simulink model "dualSpinCSSimulink"  (R2022a)
settings: Solver=VariableStepAuto  StartTime=0.0  StopTime=200  RelTol=1e-3
values from neighbouring files (symbols this model uses):
  alpha = 0.9    [dualSpinControlSystem.m]
  h_dot = 0    [dualSpinControlSystem.m]
  h_s = I_B * w_B    [dualSpinControlSystem.m]
  Ixx = 44451.50    (= 44451.5)    [dualSpinControlSystem.m]    (also in nonlinear_linear.m = interiaVector(1); singleSpinSystem.m)
  Iyy = 45161.45    [dualSpinControlSystem.m]    (also in nonlinear_linear.m = interiaVector(2); singleSpinSystem.m)
  Izz = 44017.00    (= 44017)    [dualSpinControlSystem.m]    (also in nonlinear_linear.m = interiaVector(3); singleSpinSystem.m)
  kd = 1.2    [dualSpinControlSystem.m]
  kd_p = 2 * Iyy * zeta_pitch * wN_pitch    [dualSpinControlSystem.m]
  kg = 3 * w_0_b2^2 * (Ixx-Izz)    [dualSpinControlSystem.m]
  kp = 3    [dualSpinControlSystem.m]
  kp_p = wN_pitch^2*Iyy - 3*w_0_b2^2 * (Ixx - Izz)    [dualSpinControlSystem.m]
  T = 5    [dualSpinControlSystem.m]
  tC_x = 0    [dualSpinControlSystem.m]
  tC_y = 0    [dualSpinControlSystem.m]
  tC_z = 0    [dualSpinControlSystem.m]
  tD_x = 1E-5    (= 1e-05)    [dualSpinControlSystem.m]
  tD_y = 1E-5    (= 1e-05)    [dualSpinControlSystem.m]
  tD_z = 1E-5    (= 1e-05)    [dualSpinControlSystem.m]
  w_0_b2 = sqrt(mu/R_c^3)    [dualSpinControlSystem.m]
undefined symbols (not defined in the file or in its folder): ki
settings Model: Creator=micha  LastModifiedBy=micha

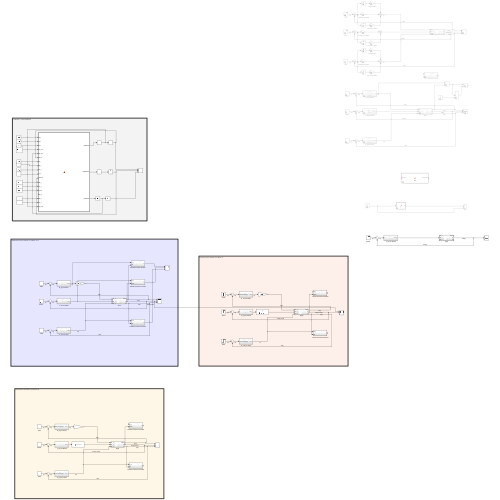
[thumbnail: Simulink's stored preview of the top-level diagram]
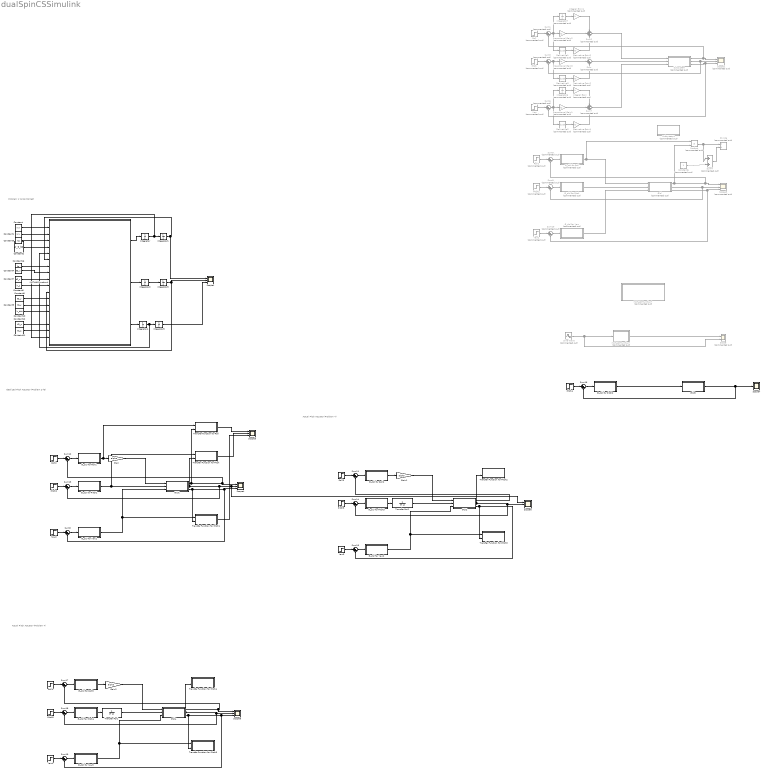
== system dualSpinCSSimulink ==
  note: Problem 1 (Uncontrolled)
  note: Actual Pitch Actuator (Problem 4)
  note: Idealized Pitch Actuator (Problem 2+3)
  note: Actual Pitch Actuator (Problem 4)
  Constant : Constant  Value=Ixx
  Constant1 : Constant  Value=Iyy
  Constant10 : Constant  Value=h_dot
  Constant11 : Constant  Value=tC_z
  Constant12 : Constant  Value=tD_z
  Constant16 : Constant  Value=kg
  Constant2 : Constant  Value=w_0_b2
  Constant3 : Constant  Value=Izz
  Constant4 : Constant  Value=tD_x
  Constant5 : Constant  Value=h_s
  Constant6 : Constant  Commented=on
  Constant7 : Constant  Value=tC_x
  Constant8 : Constant  Value=tD_y
  Constant9 : Constant  Value=tC_y
  Derivative Gain1 : Gain  Commented=on  Gain=kd
  Derivative Gain2 : Gain  Commented=on  Gain=kd
  Derivative Gain3 : Gain  Commented=on  Gain=kd
  Derivative1 : Derivative  Commented=on
  Derivative2 : Derivative  Commented=on
  Derivative3 : Derivative  Commented=on
  Divide : Product  Commented=on  Inputs=*/
  G(s) : Subsystem  Commented=on
  G(s)1 : Subsystem
  G(s)2 : Subsystem
  G(s)3 : Subsystem
  G(s)4 : Subsystem
  G_c(s) for Pitch : Subsystem  Commented=on
  G_c(s) for Pitch1 : Subsystem
  G_c(s) for Pitch2 : Subsystem
  G_c(s) for Pitch3 : Subsystem
  G_c(s) for Pitch4 : Subsystem
  G_c(s) for Roll : Subsystem  Commented=on
  G_c(s) for Roll1 : Subsystem
  G_c(s) for Roll2 : Subsystem
  G_c(s) for Roll3 : Subsystem
  G_c(s) for Yaw : Subsystem  Commented=on
  G_c(s) for Yaw1 : Subsystem
  G_c(s) for Yaw2 : Subsystem
  G_c(s) for Yaw3 : Subsystem
  Gain : Gain  Gain=alpha
  Gain1 : Gain  Gain=alpha
  Gain2 : Gain  Gain=alpha
  Integral Gain : Gain  Commented=on  Gain=ki
  Integral Gain1 : Gain  Commented=on  Gain=ki
  Integrator{,1..5} (6 alike) : Integrator
  Integrator6 : Integrator  Commented=on
  Integrator7 : Integrator  Commented=on
  MATLAB Function1 : MATLAB Function  Commented=on  TreatAsAtomicUnit=on
  MATLAB Function2 : MATLAB Function  Commented=on  TreatAsAtomicUnit=on
  MATLAB Function4 : MATLAB Function  TreatAsAtomicUnit=on
  Pitch : Step  Commented=on  SampleTime=0
  Pitch1 : Step  Commented=on  SampleTime=0
  Pitch{2..5} (4 alike) : Step  SampleTime=0
  Product : Product  Commented=on
  Proportional Gain1 : Gain  Commented=on  Gain=kp
  Proportional Gain2 : Gain  Commented=on  Gain=kp
  Proportional Gain3 : Gain  Commented=on  Gain=kp
  Roll : Step  Commented=on  SampleTime=0
  Roll1 : Step  Commented=on  SampleTime=0
  Roll2 : Step  SampleTime=0
  Roll3 : Step  SampleTime=0
  Roll4 : Step  SampleTime=0
  Scope : Scope  Commented=on  NumInputPorts=2
  Scope{1,4..8} (6 alike) : Scope  NumInputPorts=3
  Scope2 : Scope  Commented=on  NumInputPorts=3
  Scope3 : Scope  Commented=on  NumInputPorts=3
  Sine Wave : Sin  Commented=on  SampleTime=0
  Subsystem : Subsystem  Commented=on
  Subsystem1 : Subsystem  Commented=on
  Sum : Sum  Commented=on  Inputs=|++
  Sum{1,3,5..6,9..10} (6 alike) : Sum  Commented=on  Inputs=|+-
  Sum{8,11..19} (10 alike) : Sum  Inputs=|+-
  Sum2 : Sum  Commented=on  Inputs=+++
  Sum4 : Sum  Commented=on  Inputs=|++
  Sum7 : Sum  Commented=on  Inputs=+++
  Transfer Fcn1 : TransferFcn  Denominator=[T 1]
  Transfer Fcn2 : TransferFcn  Denominator=[T 1]
  Transfer Function for Pitch : Subsystem
  Transfer Function for Pitch1 : Subsystem
  Transfer Function for Pitch2 : Subsystem
  Transfer Function for Pitch3 : Subsystem
  Transfer Function for Pitch4 : Subsystem
  Transfer Function for Pitch5 : Subsystem
  "Transfer Function for Roll " : Subsystem
  Yaw : Step  Commented=on  SampleTime=0
  Yaw1 : Step  Commented=on  SampleTime=0
  Yaw2 : Step  SampleTime=0
  Yaw3 : Step  SampleTime=0
  Yaw4 : Step  SampleTime=0
  wires:
  MATLAB Function1/1(y) -> Scope/1
  Sine Wave/1 -> Scope/2, MATLAB Function1/1(u)
  MATLAB Function4/1(phiDotDot) -> Integrator/1
  Integrator/1 -> MATLAB Function4/18(phi_dot), Integrator1/1
  Constant/1 -> MATLAB Function4/1(Ixx)
  Constant1/1 -> MATLAB Function4/2(Iyy)
  Constant3/1 -> MATLAB Function4/3(Izz)
  Constant16/1 -> MATLAB Function4/7(kg)
  Constant4/1 -> MATLAB Function4/8(tD_x)
  Constant7/1 -> MATLAB Function4/9(tC_x)
  Constant2/1 -> MATLAB Function4/4(w_0_b2)
  Constant5/1 -> MATLAB Function4/10(h_s)
  Constant8/1 -> MATLAB Function4/12(tD_y)
  Constant9/1 -> MATLAB Function4/13(tC_y)
  Constant10/1 -> MATLAB Function4/14(h_dot)
  Constant12/1 -> MATLAB Function4/16(tD_z)
  Constant11/1 -> MATLAB Function4/17(tC_z)
  Integrator1/1 -> Scope1/1, MATLAB Function4/6(phi_0)
  MATLAB Function4/2(thetaDotDot) -> Integrator2/1
  Integrator2/1 -> Integrator3/1
  Integrator3/1 -> Scope1/2, MATLAB Function4/11(theta_0)
  Integrator4/1 -> MATLAB Function4/5(psi_dot), Integrator5/1
  MATLAB Function4/3(psiDotDot) -> Integrator4/1
  Integrator5/1 -> Scope1/3
  Proportional Gain1/1 -> Sum7/2
  Integrator6/1 -> Integral Gain/1
  Derivative2/1 -> Derivative Gain1/1
  Subsystem/3(Out3) -> Scope2/3, Sum6/2  "psi(t)"
  Yaw/1 -> Sum6/1  "u(t)"
  Sum6/1 -> Derivative2/1, Integrator6/1, Proportional Gain1/1  "e(t)"
  Integral Gain/1 -> Sum7/1
  Derivative Gain1/1 -> Sum7/3
  Sum1/1 -> Derivative1/1, Integrator7/1, Proportional Gain2/1  "e(t)"
  Integral Gain1/1 -> Sum2/1
  Derivative Gain2/1 -> Sum2/3
  Proportional Gain2/1 -> Sum2/2
  Integrator7/1 -> Integral Gain1/1
  Subsystem/1(Out1) -> Sum1/2, Scope2/1  "phi(t)"
  Derivative1/1 -> Derivative Gain2/1
  Roll/1 -> Sum1/1  "u(t)"
  Sum3/1 -> Derivative3/1, Proportional Gain3/1  "e(t)"
  Derivative Gain3/1 -> Sum/2
  Subsystem/2(Out2) -> Sum3/2, Scope2/2  "theta(t)"
  Derivative3/1 -> Derivative Gain3/1
  Pitch/1 -> Sum3/1  "u(t)"
  Proportional Gain3/1 -> Sum/1
  Sum7/1 -> Subsystem/3(tC_z)  "v(t)"
  Sum2/1 -> Subsystem/1(tC_x)  "v(t)"
  Sum/1 -> Subsystem/2(tC_y)
  G_c(s) for Roll/1(Out1) -> Product/1, G(s)/1(tC_x)  "v(t)"
  Sum9/1 -> G_c(s) for Pitch/1(In1)  "e(t)"
  G_c(s) for Yaw/1(tC_z) -> G(s)/3(tC_z)  "v(t)"
  G(s)/2(Out2) -> Sum9/2, Scope3/2  "theta(t)"
  Sum10/1 -> G_c(s) for Yaw/1(In1)  "e(t)"
  Roll1/1 -> Sum5/1  "u(t)"
  G(s)/3(Out3) -> Scope3/3, Sum10/2  "psi(t)"
  Pitch1/1 -> Sum9/1  "u(t)"
  G(s)/1(Out1) -> Product/2, Sum5/2, Scope3/1  "phi(t)"
  Yaw1/1 -> Sum10/1  "u(t)"
  G_c(s) for Pitch/1(tC_y) -> G(s)/2(tC_y)
  Sum5/1 -> G_c(s) for Roll/1(In1)  "e(t)"
  Product/1 -> Sum4/1, Divide/1
  Constant6/1 -> Sum4/2
  Sum4/1 -> Divide/2
  Sum8/1 -> G_c(s) for Yaw1/1(In1)  "e(t)"
  G_c(s) for Yaw1/1(tC_z) -> G(s)1/3(tC_z), Transfer Function for Pitch1/1(tC_z)  "v(t)"
  Yaw2/1 -> Sum8/1  "u(t)"
  G(s)1/1(Input) -> "Transfer Function for Roll "/2(phi), Scope4/1, Sum12/2  "phi(t)"
  Pitch2/1 -> Sum13/1  "u(t)"
  G(s)1/3(Out3) -> Transfer Function for Pitch1/2(psi), Sum8/2, Scope4/3  "psi(t)"
  Roll2/1 -> Sum12/1  "u(t)"
  G(s)1/2(Out2) -> Transfer Function for Pitch/2(theta), Sum13/2, Scope6/1, Scope4/2  "theta(t) Ideal"
  Sum13/1 -> G_c(s) for Pitch1/1(In1)  "e(t)"
  Sum12/1 -> G_c(s) for Roll1/1(In1)  "e(t)"
  G_c(s) for Roll1/1(tC_x) -> Gain/1, "Transfer Function for Roll "/1(tC_x)  "v(t)"
  G_c(s) for Pitch1/1(tC_y) -> Transfer Function for Pitch/1(tC_y), G(s)1/2(tC_y)
  "Transfer Function for Roll "/1(Out1) -> Scope5/1
  Transfer Function for Pitch/1(Out1) -> Scope5/2
  Transfer Function for Pitch1/1(Out1) -> Scope5/3
  Gain/1 -> G(s)1/1(tC_x)
  Gain1/1 -> G(s)2/1(tC_x)
  Sum14/1 -> G_c(s) for Pitch3/1(In1)  "e(t)"
  G_c(s) for Roll2/1(tC_x) -> Gain1/1  "v(t)"
  Yaw3/1 -> Sum15/1  "u(t)"
  G(s)2/2(Out2) -> Transfer Function for Pitch2/2(theta), Scope6/2, Sum14/2  "theta(t) actual"
  Pitch3/1 -> Sum14/1  "u(t)"
  Sum11/1 -> G_c(s) for Roll2/1(Roll Command)  "e(t)"
  Roll3/1 -> Sum11/1  "u(t)"
  Sum15/1 -> G_c(s) for Yaw2/1(Yaw Command)  "e(t)"
  G(s)2/1(Input) -> Sum11/2  "phi(t)"
  G(s)2/3(Out3) -> Transfer Function for Pitch3/2(psi), Sum15/2  "psi(t)"
  G_c(s) for Yaw2/1(tC_z) -> G(s)2/3(tC_z), Transfer Function for Pitch3/1(tC_z)  "v(t)"
  G_c(s) for Pitch3/1(tC_y) -> Transfer Fcn2/1
  Transfer Fcn2/1 -> G(s)2/2(tC_y)
  Sum16/1 -> G_c(s) for Pitch2/1(In1)  "e(t)"
  G(s)3/2(Out2) -> Sum16/2, Scope7/2  "theta(t)"
  G_c(s) for Pitch2/1(tC_y) -> G(s)3/2(tC_y)
  Pitch4/1 -> Sum16/1  "u(t)"
  Transfer Fcn1/1 -> G(s)4/2(tC_y)
  G_c(s) for Roll3/1(tC_x) -> Gain2/1  "v(t)"
  G_c(s) for Yaw3/1(tC_z) -> G(s)4/3(tC_z), Transfer Function for Pitch5/1(tC_z)  "v(t)"
  G(s)4/1(Input) -> Scope8/1, Sum17/2  "phi(t)"
  Sum17/1 -> G_c(s) for Roll3/1(Roll Command)  "e(t)"
  G_c(s) for Pitch4/1(tC_y) -> Transfer Fcn1/1
  Sum19/1 -> G_c(s) for Yaw3/1(Yaw Command)  "e(t)"
  Roll4/1 -> Sum17/1  "u(t)"
  G(s)4/2(Out2) -> Transfer Function for Pitch4/2(theta), Scope8/2, Sum18/2  "theta(t) actual"
  Yaw4/1 -> Sum19/1  "u(t)"
  G(s)4/3(Out3) -> Transfer Function for Pitch5/2(psi), Scope8/3, Sum19/2  "psi(t)"
  Pitch5/1 -> Sum18/1  "u(t)"
  Sum18/1 -> G_c(s) for Pitch4/1(In1)  "e(t)"
  Gain2/1 -> G(s)4/1(tC_x)

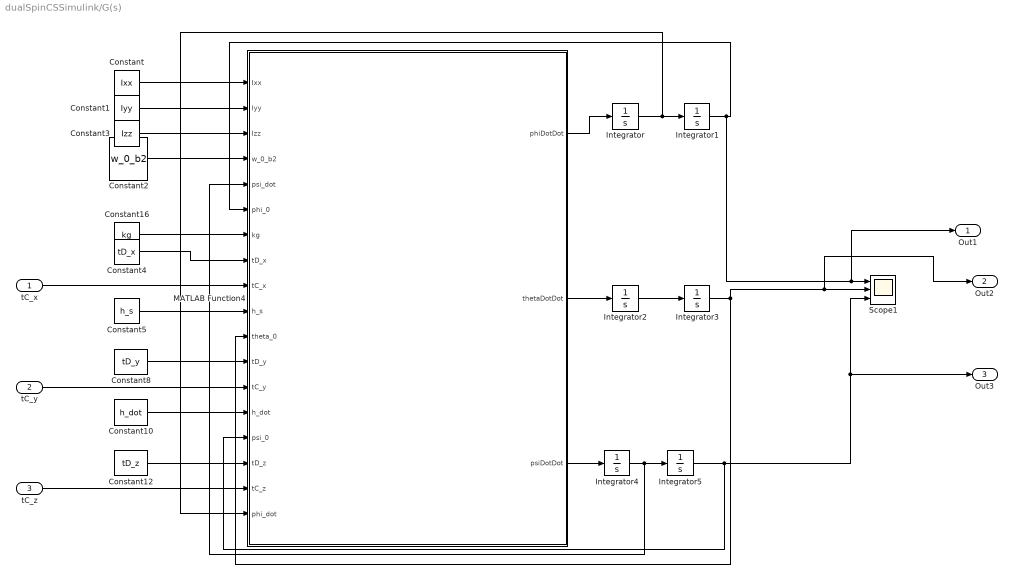
== system dualSpinCSSimulink/G(s) ==
  tC_x : Inport
  tC_y : Inport  Port=2
  tC_z : Inport  Port=3
  Constant : Constant  Value=Ixx
  Constant1 : Constant  Value=Iyy
  Constant10 : Constant  Value=h_dot
  Constant12 : Constant  Value=tD_z
  Constant16 : Constant  Value=kg
  Constant2 : Constant  Value=w_0_b2
  Constant3 : Constant  Value=Izz
  Constant4 : Constant  Value=tD_x
  Constant5 : Constant  Value=h_s
  Constant8 : Constant  Value=tD_y
  Integrator{,1..5} (6 alike) : Integrator
  MATLAB Function4 : MATLAB Function  TreatAsAtomicUnit=on
  Scope1 : Scope  NumInputPorts=3
  Out1 : Outport
  Out2 : Outport  Port=2
  Out3 : Outport  Port=3
  wires:
  tC_z/1 -> MATLAB Function4/17(tC_z)
  MATLAB Function4/2(thetaDotDot) -> Integrator2/1
  MATLAB Function4/3(psiDotDot) -> Integrator4/1
  Integrator4/1 -> MATLAB Function4/5(psi_dot), Integrator5/1
  Constant2/1 -> MATLAB Function4/4(w_0_b2)
  Constant10/1 -> MATLAB Function4/14(h_dot)
  Integrator5/1 -> MATLAB Function4/15(psi_0), Scope1/3, Out3/1
  Integrator2/1 -> Integrator3/1
  Constant/1 -> MATLAB Function4/1(Ixx)
  tC_y/1 -> MATLAB Function4/13(tC_y)
  Integrator1/1 -> Out1/1, Scope1/1, MATLAB Function4/6(phi_0)
  Constant1/1 -> MATLAB Function4/2(Iyy)
  Constant12/1 -> MATLAB Function4/16(tD_z)
  Constant16/1 -> MATLAB Function4/7(kg)
  MATLAB Function4/1(phiDotDot) -> Integrator/1
  Integrator/1 -> MATLAB Function4/18(phi_dot), Integrator1/1
  tC_x/1 -> MATLAB Function4/9(tC_x)
  Constant4/1 -> MATLAB Function4/8(tD_x)
  Constant8/1 -> MATLAB Function4/12(tD_y)
  Integrator3/1 -> Out2/1, Scope1/2, MATLAB Function4/11(theta_0)
  Constant3/1 -> MATLAB Function4/3(Izz)
  Constant5/1 -> MATLAB Function4/10(h_s)

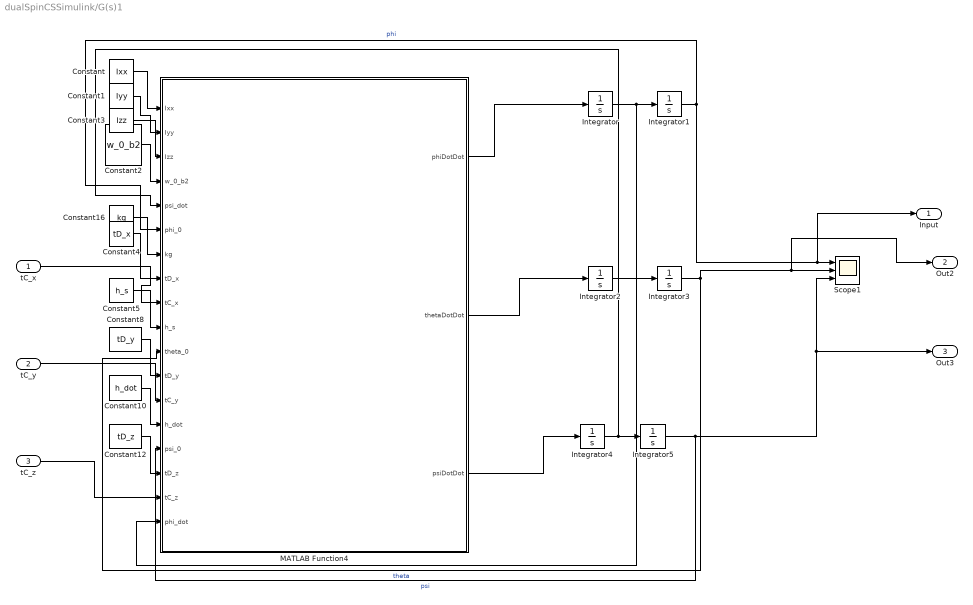
== system dualSpinCSSimulink/G(s)1 ==
  tC_x : Inport
  tC_y : Inport  Port=2
  tC_z : Inport  Port=3
  Constant : Constant  Value=Ixx
  Constant1 : Constant  Value=Iyy
  Constant10 : Constant  Value=h_dot
  Constant12 : Constant  Value=tD_z
  Constant16 : Constant  Value=kg
  Constant2 : Constant  Value=w_0_b2
  Constant3 : Constant  Value=Izz
  Constant4 : Constant  Value=tD_x
  Constant5 : Constant  Value=h_s
  Constant8 : Constant  Value=tD_y
  Integrator{,1..5} (6 alike) : Integrator
  MATLAB Function4 : MATLAB Function  TreatAsAtomicUnit=on
  Scope1 : Scope  NumInputPorts=3
  Input : Outport
  Out2 : Outport  Port=2
  Out3 : Outport  Port=3
  wires:
  tC_z/1 -> MATLAB Function4/17(tC_z)
  MATLAB Function4/2(thetaDotDot) -> Integrator2/1
  MATLAB Function4/3(psiDotDot) -> Integrator4/1
  Integrator4/1 -> MATLAB Function4/5(psi_dot), Integrator5/1
  Constant2/1 -> MATLAB Function4/4(w_0_b2)
  Constant10/1 -> MATLAB Function4/14(h_dot)
  Integrator5/1 -> MATLAB Function4/15(psi_0), Scope1/3, Out3/1  "psi"
  Integrator2/1 -> Integrator3/1
  Constant/1 -> MATLAB Function4/1(Ixx)
  tC_y/1 -> MATLAB Function4/13(tC_y)
  Integrator1/1 -> Input/1, Scope1/1, MATLAB Function4/6(phi_0)  "phi"
  Constant1/1 -> MATLAB Function4/2(Iyy)
  Constant12/1 -> MATLAB Function4/16(tD_z)
  Constant16/1 -> MATLAB Function4/7(kg)
  MATLAB Function4/1(phiDotDot) -> Integrator/1
  Integrator/1 -> MATLAB Function4/18(phi_dot), Integrator1/1
  tC_x/1 -> MATLAB Function4/9(tC_x)
  Constant4/1 -> MATLAB Function4/8(tD_x)
  Constant8/1 -> MATLAB Function4/12(tD_y)
  Integrator3/1 -> Out2/1, Scope1/2, MATLAB Function4/11(theta_0)  "theta"
  Constant3/1 -> MATLAB Function4/3(Izz)
  Constant5/1 -> MATLAB Function4/10(h_s)

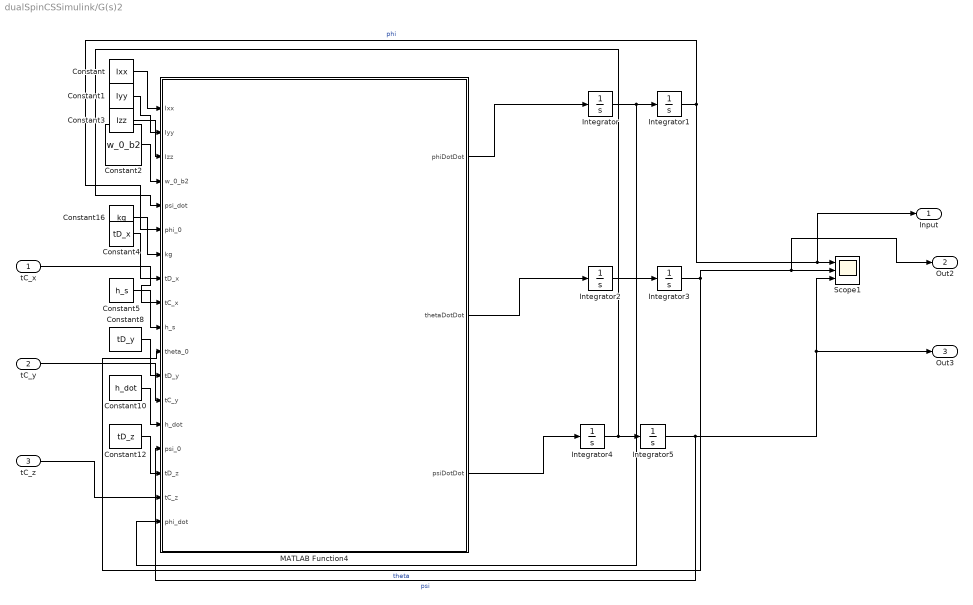
== system dualSpinCSSimulink/G(s)2 ==
  tC_x : Inport
  tC_y : Inport  Port=2
  tC_z : Inport  Port=3
  Constant : Constant  Value=Ixx
  Constant1 : Constant  Value=Iyy
  Constant10 : Constant  Value=h_dot
  Constant12 : Constant  Value=tD_z
  Constant16 : Constant  Value=kg
  Constant2 : Constant  Value=w_0_b2
  Constant3 : Constant  Value=Izz
  Constant4 : Constant  Value=tD_x
  Constant5 : Constant  Value=h_s
  Constant8 : Constant  Value=tD_y
  Integrator{,1..5} (6 alike) : Integrator
  MATLAB Function4 : MATLAB Function  TreatAsAtomicUnit=on
  Scope1 : Scope  NumInputPorts=3
  Input : Outport
  Out2 : Outport  Port=2
  Out3 : Outport  Port=3
  wires:
  tC_z/1 -> MATLAB Function4/17(tC_z)
  MATLAB Function4/2(thetaDotDot) -> Integrator2/1
  MATLAB Function4/3(psiDotDot) -> Integrator4/1
  Integrator4/1 -> MATLAB Function4/5(psi_dot), Integrator5/1
  Constant2/1 -> MATLAB Function4/4(w_0_b2)
  Constant10/1 -> MATLAB Function4/14(h_dot)
  Integrator5/1 -> MATLAB Function4/15(psi_0), Scope1/3, Out3/1  "psi"
  Integrator2/1 -> Integrator3/1
  Constant/1 -> MATLAB Function4/1(Ixx)
  tC_y/1 -> MATLAB Function4/13(tC_y)
  Integrator1/1 -> Input/1, Scope1/1, MATLAB Function4/6(phi_0)  "phi"
  Constant1/1 -> MATLAB Function4/2(Iyy)
  Constant12/1 -> MATLAB Function4/16(tD_z)
  Constant16/1 -> MATLAB Function4/7(kg)
  MATLAB Function4/1(phiDotDot) -> Integrator/1
  Integrator/1 -> MATLAB Function4/18(phi_dot), Integrator1/1
  tC_x/1 -> MATLAB Function4/9(tC_x)
  Constant4/1 -> MATLAB Function4/8(tD_x)
  Constant8/1 -> MATLAB Function4/12(tD_y)
  Integrator3/1 -> Out2/1, Scope1/2, MATLAB Function4/11(theta_0)  "theta"
  Constant3/1 -> MATLAB Function4/3(Izz)
  Constant5/1 -> MATLAB Function4/10(h_s)

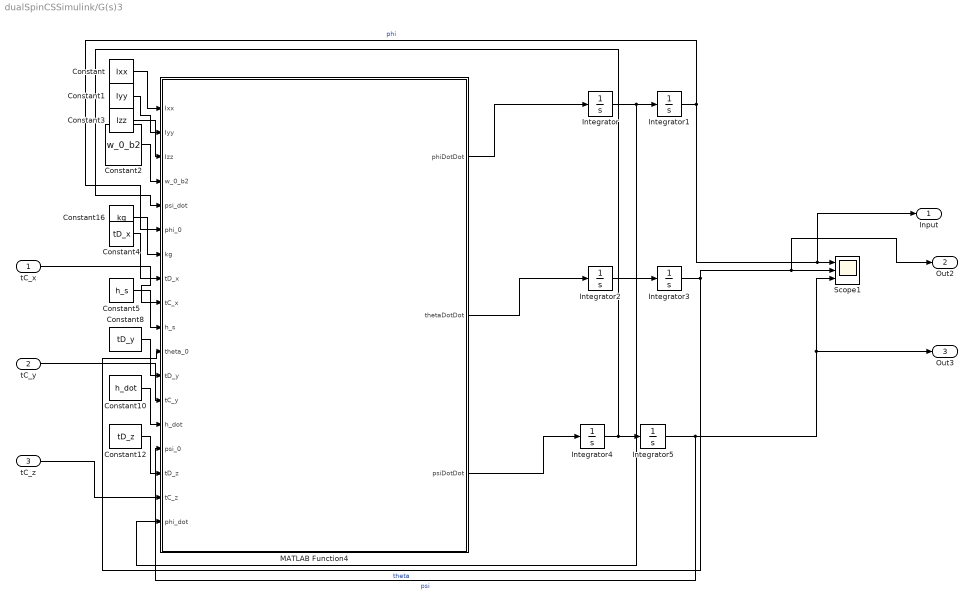
== system dualSpinCSSimulink/G(s)3 ==
  tC_x : Inport
  tC_y : Inport  Port=2
  tC_z : Inport  Port=3
  Constant : Constant  Value=Ixx
  Constant1 : Constant  Value=Iyy
  Constant10 : Constant  Value=h_dot
  Constant12 : Constant  Value=tD_z
  Constant16 : Constant  Value=kg
  Constant2 : Constant  Value=w_0_b2
  Constant3 : Constant  Value=Izz
  Constant4 : Constant  Value=tD_x
  Constant5 : Constant  Value=h_s
  Constant8 : Constant  Value=tD_y
  Integrator{,1..5} (6 alike) : Integrator
  MATLAB Function4 : MATLAB Function  TreatAsAtomicUnit=on
  Scope1 : Scope  NumInputPorts=3
  Input : Outport
  Out2 : Outport  Port=2
  Out3 : Outport  Port=3
  wires:
  tC_z/1 -> MATLAB Function4/17(tC_z)
  MATLAB Function4/2(thetaDotDot) -> Integrator2/1
  MATLAB Function4/3(psiDotDot) -> Integrator4/1
  Integrator4/1 -> MATLAB Function4/5(psi_dot), Integrator5/1
  Constant2/1 -> MATLAB Function4/4(w_0_b2)
  Constant10/1 -> MATLAB Function4/14(h_dot)
  Integrator5/1 -> MATLAB Function4/15(psi_0), Scope1/3, Out3/1  "psi"
  Integrator2/1 -> Integrator3/1
  Constant/1 -> MATLAB Function4/1(Ixx)
  tC_y/1 -> MATLAB Function4/13(tC_y)
  Integrator1/1 -> Input/1, Scope1/1, MATLAB Function4/6(phi_0)  "phi"
  Constant1/1 -> MATLAB Function4/2(Iyy)
  Constant12/1 -> MATLAB Function4/16(tD_z)
  Constant16/1 -> MATLAB Function4/7(kg)
  MATLAB Function4/1(phiDotDot) -> Integrator/1
  Integrator/1 -> MATLAB Function4/18(phi_dot), Integrator1/1
  tC_x/1 -> MATLAB Function4/9(tC_x)
  Constant4/1 -> MATLAB Function4/8(tD_x)
  Constant8/1 -> MATLAB Function4/12(tD_y)
  Integrator3/1 -> Out2/1, Scope1/2, MATLAB Function4/11(theta_0)  "theta"
  Constant3/1 -> MATLAB Function4/3(Izz)
  Constant5/1 -> MATLAB Function4/10(h_s)

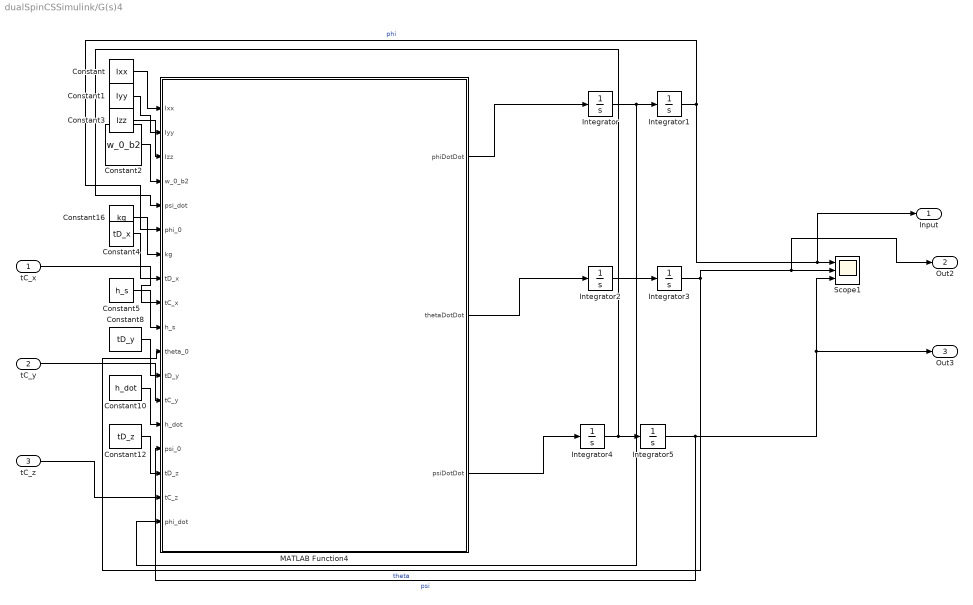
== system dualSpinCSSimulink/G(s)4 ==
  tC_x : Inport
  tC_y : Inport  Port=2
  tC_z : Inport  Port=3
  Constant : Constant  Value=Ixx
  Constant1 : Constant  Value=Iyy
  Constant10 : Constant  Value=h_dot
  Constant12 : Constant  Value=tD_z
  Constant16 : Constant  Value=kg
  Constant2 : Constant  Value=w_0_b2
  Constant3 : Constant  Value=Izz
  Constant4 : Constant  Value=tD_x
  Constant5 : Constant  Value=h_s
  Constant8 : Constant  Value=tD_y
  Integrator{,1..5} (6 alike) : Integrator
  MATLAB Function4 : MATLAB Function  TreatAsAtomicUnit=on
  Scope1 : Scope  NumInputPorts=3
  Input : Outport
  Out2 : Outport  Port=2
  Out3 : Outport  Port=3
  wires:
  tC_z/1 -> MATLAB Function4/17(tC_z)
  MATLAB Function4/2(thetaDotDot) -> Integrator2/1
  MATLAB Function4/3(psiDotDot) -> Integrator4/1
  Integrator4/1 -> MATLAB Function4/5(psi_dot), Integrator5/1
  Constant2/1 -> MATLAB Function4/4(w_0_b2)
  Constant10/1 -> MATLAB Function4/14(h_dot)
  Integrator5/1 -> MATLAB Function4/15(psi_0), Scope1/3, Out3/1  "psi"
  Integrator2/1 -> Integrator3/1
  Constant/1 -> MATLAB Function4/1(Ixx)
  tC_y/1 -> MATLAB Function4/13(tC_y)
  Integrator1/1 -> Input/1, Scope1/1, MATLAB Function4/6(phi_0)  "phi"
  Constant1/1 -> MATLAB Function4/2(Iyy)
  Constant12/1 -> MATLAB Function4/16(tD_z)
  Constant16/1 -> MATLAB Function4/7(kg)
  MATLAB Function4/1(phiDotDot) -> Integrator/1
  Integrator/1 -> MATLAB Function4/18(phi_dot), Integrator1/1
  tC_x/1 -> MATLAB Function4/9(tC_x)
  Constant4/1 -> MATLAB Function4/8(tD_x)
  Constant8/1 -> MATLAB Function4/12(tD_y)
  Integrator3/1 -> Out2/1, Scope1/2, MATLAB Function4/11(theta_0)  "theta"
  Constant3/1 -> MATLAB Function4/3(Izz)
  Constant5/1 -> MATLAB Function4/10(h_s)

== system dualSpinCSSimulink/G_c(s) for Pitch ==
  In1 : Inport
  Derivative Gain6 : Gain  Gain=kd
  Derivative6 : Derivative
  Proportional Gain6 : Gain  Gain=kp
  Sum : Sum  Inputs=|++
  tC_y : Outport
  wires:
  Derivative6/1 -> Derivative Gain6/1
  Proportional Gain6/1 -> Sum/1
  In1/1 -> Derivative6/1, Proportional Gain6/1  "e(t)"
  Derivative Gain6/1 -> Sum/2
  Sum/1 -> tC_y/1

== system dualSpinCSSimulink/G_c(s) for Pitch1 ==
  In1 : Inport
  Derivative Gain6 : Gain  Gain=kd_p
  Derivative6 : Derivative
  Proportional Gain6 : Gain  Gain=kp_p
  Sum : Sum  Inputs=|++
  tC_y : Outport
  wires:
  Derivative6/1 -> Derivative Gain6/1
  Proportional Gain6/1 -> Sum/1
  In1/1 -> Derivative6/1, Proportional Gain6/1  "e(t)"
  Derivative Gain6/1 -> Sum/2
  Sum/1 -> tC_y/1

== system dualSpinCSSimulink/G_c(s) for Pitch2 ==
  In1 : Inport
  Derivative Gain6 : Gain  Gain=kd_p
  Derivative6 : Derivative
  Proportional Gain6 : Gain  Gain=kp_p
  Sum : Sum  Inputs=|++
  tC_y : Outport
  wires:
  Derivative6/1 -> Derivative Gain6/1
  Proportional Gain6/1 -> Sum/1
  In1/1 -> Derivative6/1, Proportional Gain6/1  "e(t)"
  Derivative Gain6/1 -> Sum/2
  Sum/1 -> tC_y/1

== system dualSpinCSSimulink/G_c(s) for Pitch3 ==
  In1 : Inport
  Derivative Gain6 : Gain  Gain=kd_p
  Derivative6 : Derivative
  Proportional Gain6 : Gain  Gain=kp_p
  Sum : Sum  Inputs=|++
  tC_y : Outport
  wires:
  Derivative6/1 -> Derivative Gain6/1
  Proportional Gain6/1 -> Sum/1
  In1/1 -> Derivative6/1, Proportional Gain6/1  "e(t)"
  Derivative Gain6/1 -> Sum/2
  Sum/1 -> tC_y/1

== system dualSpinCSSimulink/G_c(s) for Pitch4 ==
  In1 : Inport
  Derivative Gain6 : Gain  Gain=kd_p
  Derivative6 : Derivative
  Proportional Gain6 : Gain  Gain=kp_p
  Sum : Sum  Inputs=|++
  tC_y : Outport
  wires:
  Derivative6/1 -> Derivative Gain6/1
  Proportional Gain6/1 -> Sum/1
  In1/1 -> Derivative6/1, Proportional Gain6/1  "e(t)"
  Derivative Gain6/1 -> Sum/2
  Sum/1 -> tC_y/1

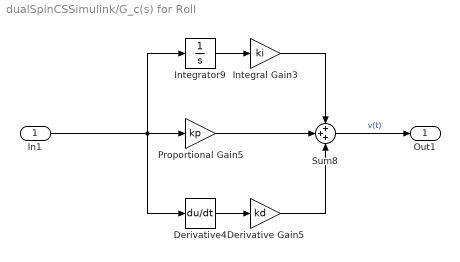
== system dualSpinCSSimulink/G_c(s) for Roll ==
  In1 : Inport
  Derivative Gain5 : Gain  Gain=kd
  Derivative4 : Derivative
  Integral Gain3 : Gain  Gain=ki
  Integrator9 : Integrator
  Proportional Gain5 : Gain  Gain=kp
  Sum8 : Sum  Inputs=+++
  Out1 : Outport
  wires:
  Derivative Gain5/1 -> Sum8/3
  Integral Gain3/1 -> Sum8/1
  Derivative4/1 -> Derivative Gain5/1
  Integrator9/1 -> Integral Gain3/1
  Proportional Gain5/1 -> Sum8/2
  In1/1 -> Derivative4/1, Integrator9/1, Proportional Gain5/1
  Sum8/1 -> Out1/1  "v(t)"

== system dualSpinCSSimulink/G_c(s) for Roll1 ==
  In1 : Inport
  Derivative Gain5 : Gain  Gain=kd
  Derivative4 : Derivative
  Proportional Gain5 : Gain  Gain=kp
  Sum : Sum  Inputs=|++
  tC_x : Outport
  wires:
  Derivative Gain5/1 -> Sum/2
  Derivative4/1 -> Derivative Gain5/1
  Proportional Gain5/1 -> Sum/1
  In1/1 -> Derivative4/1, Proportional Gain5/1
  Sum/1 -> tC_x/1  "v(t)"

== system dualSpinCSSimulink/G_c(s) for Roll2 ==
  Roll Command : Inport
  Derivative Gain : Gain  Gain=kd
  Derivative4 : Derivative
  Proportional Gain : Gain  Gain=kp
  Sum : Sum  Inputs=|++
  tC_x : Outport
  wires:
  Derivative Gain/1 -> Sum/2
  Derivative4/1 -> Derivative Gain/1
  Proportional Gain/1 -> Sum/1
  Roll Command/1 -> Derivative4/1, Proportional Gain/1
  Sum/1 -> tC_x/1

== system dualSpinCSSimulink/G_c(s) for Roll3 ==
  Roll Command : Inport
  Derivative Gain : Gain  Gain=kd
  Derivative4 : Derivative
  Proportional Gain : Gain  Gain=kp
  Sum : Sum  Inputs=|++
  tC_x : Outport
  wires:
  Derivative Gain/1 -> Sum/2
  Derivative4/1 -> Derivative Gain/1
  Proportional Gain/1 -> Sum/1
  Roll Command/1 -> Derivative4/1, Proportional Gain/1
  Sum/1 -> tC_x/1

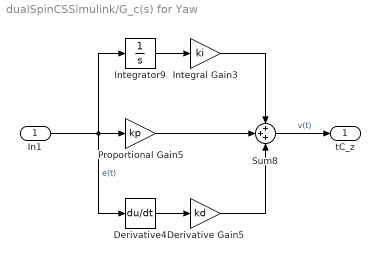
== system dualSpinCSSimulink/G_c(s) for Yaw ==
  In1 : Inport
  Derivative Gain5 : Gain  Gain=kd
  Derivative4 : Derivative
  Integral Gain3 : Gain  Gain=ki
  Integrator9 : Integrator
  Proportional Gain5 : Gain  Gain=kp
  Sum8 : Sum  Inputs=+++
  tC_z : Outport
  wires:
  Derivative Gain5/1 -> Sum8/3
  In1/1 -> Derivative4/1, Integrator9/1, Proportional Gain5/1  "e(t)"
  Integral Gain3/1 -> Sum8/1
  Derivative4/1 -> Derivative Gain5/1
  Integrator9/1 -> Integral Gain3/1
  Proportional Gain5/1 -> Sum8/2
  Sum8/1 -> tC_z/1  "v(t)"

== system dualSpinCSSimulink/G_c(s) for Yaw1 ==
  In1 : Inport
  Derivative Gain5 : Gain  Gain=kd
  Derivative4 : Derivative
  Proportional Gain5 : Gain  Gain=kp
  Sum : Sum  Inputs=|++
  tC_z : Outport
  wires:
  Derivative Gain5/1 -> Sum/2
  In1/1 -> Derivative4/1, Proportional Gain5/1  "e(t)"
  Derivative4/1 -> Derivative Gain5/1
  Proportional Gain5/1 -> Sum/1
  Sum/1 -> tC_z/1  "v(t)"

== system dualSpinCSSimulink/G_c(s) for Yaw2 ==
  Yaw Command : Inport
  Derivative Gain : Gain  Gain=kd
  Derivative4 : Derivative
  Proportional Gain : Gain  Gain=kp
  Sum : Sum  Inputs=|++
  tC_z : Outport
  wires:
  Derivative Gain/1 -> Sum/2
  Yaw Command/1 -> Derivative4/1, Proportional Gain/1  "e(t)"
  Derivative4/1 -> Derivative Gain/1
  Proportional Gain/1 -> Sum/1
  Sum/1 -> tC_z/1

== system dualSpinCSSimulink/G_c(s) for Yaw3 ==
  Yaw Command : Inport
  Derivative Gain : Gain  Gain=kd
  Derivative4 : Derivative
  Proportional Gain : Gain  Gain=kp
  Sum : Sum  Inputs=|++
  tC_z : Outport
  wires:
  Derivative Gain/1 -> Sum/2
  Yaw Command/1 -> Derivative4/1, Proportional Gain/1  "e(t)"
  Derivative4/1 -> Derivative Gain/1
  Proportional Gain/1 -> Sum/1
  Sum/1 -> tC_z/1

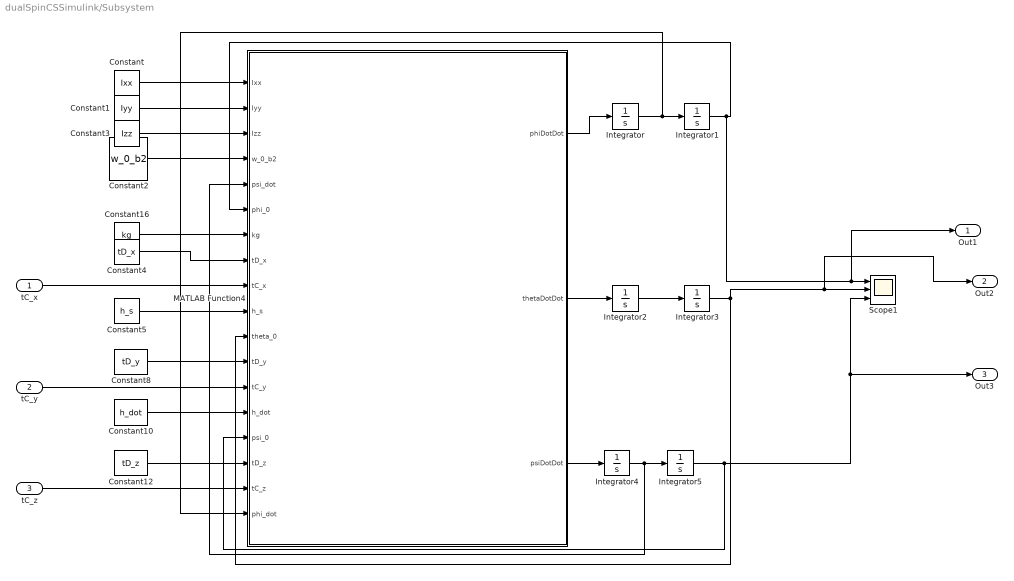
== system dualSpinCSSimulink/Subsystem ==
  tC_x : Inport
  tC_y : Inport  Port=2
  tC_z : Inport  Port=3
  Constant : Constant  Value=Ixx
  Constant1 : Constant  Value=Iyy
  Constant10 : Constant  Value=h_dot
  Constant12 : Constant  Value=tD_z
  Constant16 : Constant  Value=kg
  Constant2 : Constant  Value=w_0_b2
  Constant3 : Constant  Value=Izz
  Constant4 : Constant  Value=tD_x
  Constant5 : Constant  Value=h_s
  Constant8 : Constant  Value=tD_y
  Integrator{,1..5} (6 alike) : Integrator
  MATLAB Function4 : MATLAB Function  TreatAsAtomicUnit=on
  Scope1 : Scope  NumInputPorts=3
  Out1 : Outport
  Out2 : Outport  Port=2
  Out3 : Outport  Port=3
  wires:
  tC_z/1 -> MATLAB Function4/17(tC_z)
  MATLAB Function4/2(thetaDotDot) -> Integrator2/1
  MATLAB Function4/3(psiDotDot) -> Integrator4/1
  Integrator4/1 -> MATLAB Function4/5(psi_dot), Integrator5/1
  Constant2/1 -> MATLAB Function4/4(w_0_b2)
  Constant10/1 -> MATLAB Function4/14(h_dot)
  Integrator5/1 -> MATLAB Function4/15(psi_0), Scope1/3, Out3/1
  Integrator2/1 -> Integrator3/1
  Constant/1 -> MATLAB Function4/1(Ixx)
  tC_y/1 -> MATLAB Function4/13(tC_y)
  Integrator1/1 -> Out1/1, Scope1/1, MATLAB Function4/6(phi_0)
  Constant1/1 -> MATLAB Function4/2(Iyy)
  Constant12/1 -> MATLAB Function4/16(tD_z)
  Constant16/1 -> MATLAB Function4/7(kg)
  MATLAB Function4/1(phiDotDot) -> Integrator/1
  Integrator/1 -> MATLAB Function4/18(phi_dot), Integrator1/1
  tC_x/1 -> MATLAB Function4/9(tC_x)
  Constant4/1 -> MATLAB Function4/8(tD_x)
  Constant8/1 -> MATLAB Function4/12(tD_y)
  Integrator3/1 -> Out2/1, Scope1/2, MATLAB Function4/11(theta_0)
  Constant3/1 -> MATLAB Function4/3(Izz)
  Constant5/1 -> MATLAB Function4/10(h_s)

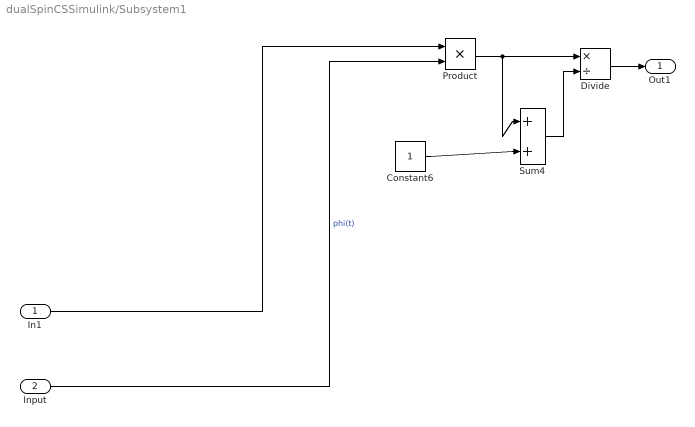
== system dualSpinCSSimulink/Subsystem1 ==
  In1 : Inport
  Input : Inport  Port=2
  Constant6 : Constant
  Divide : Product  Inputs=*/
  Product : Product
  Sum4 : Sum  Inputs=|++
  Out1 : Outport
  wires:
  Sum4/1 -> Divide/2
  Product/1 -> Sum4/1, Divide/1
  Constant6/1 -> Sum4/2
  Input/1 -> Product/2  "phi(t)"
  In1/1 -> Product/1
  Divide/1 -> Out1/1

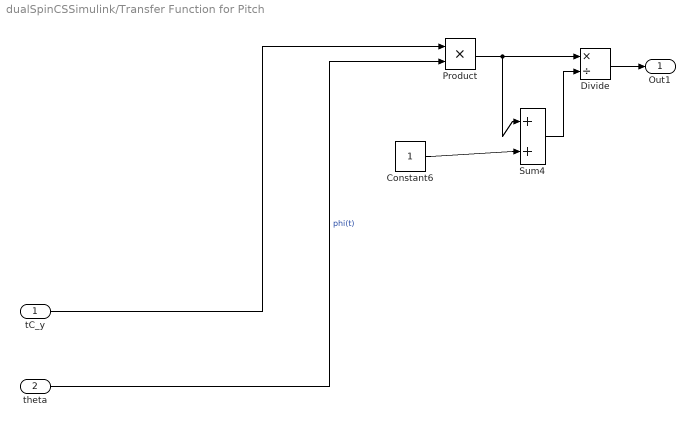
== system dualSpinCSSimulink/Transfer Function for Pitch ==
  tC_y : Inport
  theta : Inport  Port=2
  Constant6 : Constant
  Divide : Product  Inputs=*/
  Product : Product
  Sum4 : Sum  Inputs=|++
  Out1 : Outport
  wires:
  Sum4/1 -> Divide/2
  Product/1 -> Sum4/1, Divide/1
  Constant6/1 -> Sum4/2
  theta/1 -> Product/2  "phi(t)"
  tC_y/1 -> Product/1
  Divide/1 -> Out1/1

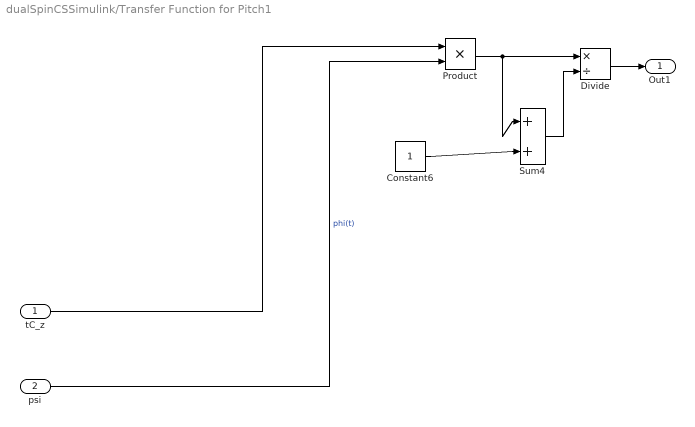
== system dualSpinCSSimulink/Transfer Function for Pitch1 ==
  tC_z : Inport
  psi : Inport  Port=2
  Constant6 : Constant
  Divide : Product  Inputs=*/
  Product : Product
  Sum4 : Sum  Inputs=|++
  Out1 : Outport
  wires:
  Divide/1 -> Out1/1
  tC_z/1 -> Product/1
  psi/1 -> Product/2  "phi(t)"
  Constant6/1 -> Sum4/2
  Product/1 -> Divide/1, Sum4/1
  Sum4/1 -> Divide/2

== system dualSpinCSSimulink/Transfer Function for Pitch2 ==
  tC_y : Inport
  theta : Inport  Port=2
  Constant6 : Constant
  Divide : Product  Inputs=*/
  Product : Product
  Sum4 : Sum  Inputs=|++
  Out1 : Outport
  wires:
  Sum4/1 -> Divide/2
  Product/1 -> Sum4/1, Divide/1
  Constant6/1 -> Sum4/2
  theta/1 -> Product/2  "phi(t)"
  tC_y/1 -> Product/1
  Divide/1 -> Out1/1

== system dualSpinCSSimulink/Transfer Function for Pitch3 ==
  tC_z : Inport
  psi : Inport  Port=2
  Constant6 : Constant
  Divide : Product  Inputs=*/
  Product : Product
  Sum4 : Sum  Inputs=|++
  Out1 : Outport
  wires:
  Divide/1 -> Out1/1
  tC_z/1 -> Product/1
  psi/1 -> Product/2  "phi(t)"
  Constant6/1 -> Sum4/2
  Product/1 -> Divide/1, Sum4/1
  Sum4/1 -> Divide/2

== system dualSpinCSSimulink/Transfer Function for Pitch4 ==
  tC_y : Inport
  theta : Inport  Port=2
  Constant6 : Constant
  Divide : Product  Inputs=*/
  Product : Product
  Sum4 : Sum  Inputs=|++
  Out1 : Outport
  wires:
  Sum4/1 -> Divide/2
  Product/1 -> Sum4/1, Divide/1
  Constant6/1 -> Sum4/2
  theta/1 -> Product/2  "phi(t)"
  tC_y/1 -> Product/1
  Divide/1 -> Out1/1

== system dualSpinCSSimulink/Transfer Function for Pitch5 ==
  tC_z : Inport
  psi : Inport  Port=2
  Constant6 : Constant
  Divide : Product  Inputs=*/
  Product : Product
  Sum4 : Sum  Inputs=|++
  Out1 : Outport
  wires:
  Divide/1 -> Out1/1
  tC_z/1 -> Product/1
  psi/1 -> Product/2  "phi(t)"
  Constant6/1 -> Sum4/2
  Product/1 -> Divide/1, Sum4/1
  Sum4/1 -> Divide/2

== system dualSpinCSSimulink/Transfer Function for Roll  ==
  tC_x : Inport
  phi : Inport  Port=2
  Constant6 : Constant
  Divide : Product  Inputs=*/
  Product : Product
  Sum4 : Sum  Inputs=|++
  Out1 : Outport
  wires:
  Sum4/1 -> Divide/2
  Product/1 -> Sum4/1, Divide/1
  Constant6/1 -> Sum4/2
  phi/1 -> Product/2  "phi(t)"
  tC_x/1 -> Product/1
  Divide/1 -> Out1/1

== matlab function dualSpinCSSimulink/G(s)1/MATLAB Function4 ==
  settings: updateMethod=CONTINUOUS
  data: Ixx input; phiDotDot output; Iyy input; Izz input; w_0_b2 input; psi_dot input; phi_0 input; kg input; tD_x input; tC_x input; h_s input; theta_0 input; tD_y input; tC_y input; h_dot input; psi_0 input; tD_z input; tC_z input; phi_dot input; thetaDotDot output; psiDotDot output
function [phiDotDot, thetaDotDot, psiDotDot] = myFunction(Ixx, Iyy, Izz, w_0_b2, psi_dot, phi_0, kg, tD_x, tC_x, h_s, theta_0, tD_y, tC_y, h_dot, psi_0, tD_z, tC_z, phi_dot)
    phiDotDot = inv(Ixx) * (((Ixx-Iyy+Izz)*w_0_b2*psi_dot) - (phi_0 *(kg+w_0_b2^2*(Ixx-Izz)))+tD_x+tC_x-h_s(2)*(phi_0*w_0_b2+psi_dot));
    thetaDotDot = inv(Iyy) * ((-kg*theta_0 + tD_y + tC_y) +h_dot);
    psiDotDot = inv(Izz)*(-1*(Ixx-Iyy+Izz)*w_0_b2*phi_dot - w_0_b2^2*psi(Iyy-Ixx) + tD_z+tC_z+h_s(2)*(phi_dot-psi_0*w_0_b2));
end

== matlab function dualSpinCSSimulink/G(s)2/MATLAB Function4 ==
  settings: updateMethod=CONTINUOUS
  data: Ixx input; phiDotDot output; Iyy input; Izz input; w_0_b2 input; psi_dot input; phi_0 input; kg input; tD_x input; tC_x input; h_s input; theta_0 input; tD_y input; tC_y input; h_dot input; psi_0 input; tD_z input; tC_z input; phi_dot input; thetaDotDot output; psiDotDot output
function [phiDotDot, thetaDotDot, psiDotDot] = myFunction(Ixx, Iyy, Izz, w_0_b2, psi_dot, phi_0, kg, tD_x, tC_x, h_s, theta_0, tD_y, tC_y, h_dot, psi_0, tD_z, tC_z, phi_dot)
    phiDotDot = inv(Ixx) * (((Ixx-Iyy+Izz)*w_0_b2*psi_dot) - (phi_0 *(kg+w_0_b2^2*(Ixx-Izz)))+tD_x+tC_x-h_s(2)*(phi_0*w_0_b2+psi_dot));
    thetaDotDot = inv(Iyy) * ((-kg*theta_0 + tD_y + tC_y) +h_dot);
    psiDotDot = inv(Izz)*(-1*(Ixx-Iyy+Izz)*w_0_b2*phi_dot - w_0_b2^2*psi(Iyy-Ixx) + tD_z+tC_z+h_s(2)*(phi_dot-psi_0*w_0_b2));
end

== matlab function dualSpinCSSimulink/G(s)3/MATLAB Function4 ==
  settings: updateMethod=CONTINUOUS
  data: Ixx input; phiDotDot output; Iyy input; Izz input; w_0_b2 input; psi_dot input; phi_0 input; kg input; tD_x input; tC_x input; h_s input; theta_0 input; tD_y input; tC_y input; h_dot input; psi_0 input; tD_z input; tC_z input; phi_dot input; thetaDotDot output; psiDotDot output
function [phiDotDot, thetaDotDot, psiDotDot] = myFunction(Ixx, Iyy, Izz, w_0_b2, psi_dot, phi_0, kg, tD_x, tC_x, h_s, theta_0, tD_y, tC_y, h_dot, psi_0, tD_z, tC_z, phi_dot)
    phiDotDot = inv(Ixx) * (((Ixx-Iyy+Izz)*w_0_b2*psi_dot) - (phi_0 *(kg+w_0_b2^2*(Ixx-Izz)))+tD_x+tC_x-h_s(2)*(phi_0*w_0_b2+psi_dot));
    thetaDotDot = inv(Iyy) * ((-kg*theta_0 + tD_y + tC_y) +h_dot);
    psiDotDot = inv(Izz)*(-1*(Ixx-Iyy+Izz)*w_0_b2*phi_dot - w_0_b2^2*psi(Iyy-Ixx) + tD_z+tC_z+h_s(2)*(phi_dot-psi_0*w_0_b2));
end

== matlab function dualSpinCSSimulink/G(s)4/MATLAB Function4 ==
  settings: updateMethod=CONTINUOUS
  data: Ixx input; phiDotDot output; Iyy input; Izz input; w_0_b2 input; psi_dot input; phi_0 input; kg input; tD_x input; tC_x input; h_s input; theta_0 input; tD_y input; tC_y input; h_dot input; psi_0 input; tD_z input; tC_z input; phi_dot input; thetaDotDot output; psiDotDot output
function [phiDotDot, thetaDotDot, psiDotDot] = myFunction(Ixx, Iyy, Izz, w_0_b2, psi_dot, phi_0, kg, tD_x, tC_x, h_s, theta_0, tD_y, tC_y, h_dot, psi_0, tD_z, tC_z, phi_dot)
    phiDotDot = inv(Ixx) * (((Ixx-Iyy+Izz)*w_0_b2*psi_dot) - (phi_0 *(kg+w_0_b2^2*(Ixx-Izz)))+tD_x+tC_x-h_s(2)*(phi_0*w_0_b2+psi_dot));
    thetaDotDot = inv(Iyy) * ((-kg*theta_0 + tD_y + tC_y) +h_dot);
    psiDotDot = inv(Izz)*(-1*(Ixx-Iyy+Izz)*w_0_b2*phi_dot - w_0_b2^2*psi(Iyy-Ixx) + tD_z+tC_z+h_s(2)*(phi_dot-psi_0*w_0_b2));
end

== matlab function dualSpinCSSimulink/MATLAB Function1 ==
  data: y output; u input
function y = fcn(u)

if u>0
    y=1;
else
    y=-1;
end

== matlab function dualSpinCSSimulink/MATLAB Function4 ==
  settings: updateMethod=CONTINUOUS
  data: Ixx input; phiDotDot output; Iyy input; Izz input; w_0_b2 input; psi_dot input; phi_0 input; kg input; tD_x input; tC_x input; h_s input; theta_0 input; tD_y input; tC_y input; h_dot input; psi_0 input; tD_z input; tC_z input; phi_dot input; thetaDotDot output; psiDotDot output
function [phiDotDot, thetaDotDot, psiDotDot] = myFunction(Ixx, Iyy, Izz, w_0_b2, psi_dot, phi_0, kg, tD_x, tC_x, h_s, theta_0, tD_y, tC_y, h_dot, psi_0, tD_z, tC_z, phi_dot)
    phiDotDot = inv(Ixx) * (((Ixx-Iyy+Izz)*w_0_b2*psi_dot) - (phi_0 *(kg+w_0_b2^2*(Ixx-Izz)))+tD_x+tC_x-h_s(2)*(phi_0*w_0_b2+psi_dot));
    thetaDotDot = inv(Iyy) * ((-kg*theta_0 + tD_y + tC_y) +h_dot);
    psiDotDot = abs(inv(Izz)*(-1*(Ixx-Iyy+Izz)*w_0_b2*phi_dot - w_0_b2^2*psi(Iyy-Ixx) + tD_z+tC_z+h_s(2)*(phi_dot-psi_0*w_0_b2)));
end

== matlab function dualSpinCSSimulink/MATLAB Function2 ==
  settings: updateMethod=CONTINUOUS
  data: unused input; phiDotDot output
function phiDotDot  = fcn(unused)

phiDotDot = inv(Ixx) * (((Ixx-Iyy+Izz)*w_0_b2*psi_dot) - (phi_0 *(kg+w_0_b2^2*(Ixx-Izz)))+tD_x+tC_x-h_s(2)*(phi_0*w_0_b2+psi_dot));
% thetaDotDot = inv(Iyy) * ((-kg*theta_0 + tD_y + tC_y) +h_dot);
% psiDotDot = inv(Izz)*(-1*(Ixx-Iyy+Izz)*w_0_b2*phi_dot - w_0_b2^2*psi(Iyy-Ixx) + tD_z+tC_z+h_s(2)*(phi_dot-psi_0*w_0_b2));



end

== matlab function dualSpinCSSimulink/Subsystem/MATLAB Function4 ==
  settings: updateMethod=CONTINUOUS
  data: Ixx input; phiDotDot output; Iyy input; Izz input; w_0_b2 input; psi_dot input; phi_0 input; kg input; tD_x input; tC_x input; h_s input; theta_0 input; tD_y input; tC_y input; h_dot input; psi_0 input; tD_z input; tC_z input; phi_dot input; thetaDotDot output; psiDotDot output
function [phiDotDot, thetaDotDot, psiDotDot] = myFunction(Ixx, Iyy, Izz, w_0_b2, psi_dot, phi_0, kg, tD_x, tC_x, h_s, theta_0, tD_y, tC_y, h_dot, psi_0, tD_z, tC_z, phi_dot)
    phiDotDot = inv(Ixx) * (((Ixx-Iyy+Izz)*w_0_b2*psi_dot) - (phi_0 *(kg+w_0_b2^2*(Ixx-Izz)))+tD_x+tC_x-h_s(2)*(phi_0*w_0_b2+psi_dot));
    thetaDotDot = inv(Iyy) * ((-kg*theta_0 + tD_y + tC_y) +h_dot);
    psiDotDot = inv(Izz)*(-1*(Ixx-Iyy+Izz)*w_0_b2*phi_dot - w_0_b2^2*psi(Iyy-Ixx) + tD_z+tC_z+h_s(2)*(phi_dot-psi_0*w_0_b2));
end

== matlab function dualSpinCSSimulink/G(s)/MATLAB Function4 ==
  settings: updateMethod=CONTINUOUS
  data: Ixx input; phiDotDot output; Iyy input; Izz input; w_0_b2 input; psi_dot input; phi_0 input; kg input; tD_x input; tC_x input; h_s input; theta_0 input; tD_y input; tC_y input; h_dot input; psi_0 input; tD_z input; tC_z input; phi_dot input; thetaDotDot output; psiDotDot output
function [phiDotDot, thetaDotDot, psiDotDot] = myFunction(Ixx, Iyy, Izz, w_0_b2, psi_dot, phi_0, kg, tD_x, tC_x, h_s, theta_0, tD_y, tC_y, h_dot, psi_0, tD_z, tC_z, phi_dot)
    phiDotDot = inv(Ixx) * (((Ixx-Iyy+Izz)*w_0_b2*psi_dot) - (phi_0 *(kg+w_0_b2^2*(Ixx-Izz)))+tD_x+tC_x-h_s(2)*(phi_0*w_0_b2+psi_dot));
    thetaDotDot = inv(Iyy) * ((-kg*theta_0 + tD_y + tC_y) +h_dot);
    psiDotDot = inv(Izz)*(-1*(Ixx-Iyy+Izz)*w_0_b2*phi_dot - w_0_b2^2*psi(Iyy-Ixx) + tD_z+tC_z+h_s(2)*(phi_dot-psi_0*w_0_b2));
end
